simulink model "PubIfChassisAHBC_MDL"  (R2020b)
settings: Solver=FixedStepDiscrete  StartTime=0.0  StopTime=10.0  FixedStep=0.02  RelTol=1e-3
settings Model: DataDictionary=AHBC.sldd  Creator=mi  LastModifiedBy=GW00204750
settings OptimizationCC: DefaultParameterBehavior=Inlined  EnhancedBackFolding=on  PassReuseOutputArgsAs=Individual arguments  ZeroExternalMemoryAtStartup=off  ZeroInternalMemoryAtStartup=off  OptimizeBlockOrder=speed  DifferentSizesBufferReuse=on  OptimizationCustomize=off  EfficientTunableParamExpr=on
settings DebuggingCC: ParameterPrecisionLossMsg=none  ParameterTunabilityLossMsg=error  SFExecutionAtInitializationDiag=none  UnderSpecifiedDimensionMsg=warning  ArithmeticOperatorsInVariantConditions=warning
settings SFSimCC: MATLABDynamicMemAlloc=off  CustomCodeUndefinedFunction=UseInterfaceOnly
settings RTWCC: Description=Embedded Coder  SystemTargetFile=ert.tlc  TemplateMakefile=ert_default_tmf  GenerateReport=on  Toolchain=Microsoft Visual C++ 2019 v16.0 | nmake (64-bit Windows)  IncludeHyperlinkInReport=on  LaunchReport=on  GenerateTraceInfo=on  GenerateTraceReport=on  GenerateTraceReportSl=on  GenerateTraceReportSf=on  GenerateTraceReportEml=on
settings CodeAppCC: ForceParamTrailComments=on  IgnoreCustomStorageClasses=off  OperatorAnnotations=on  SimulinkDataObjDesc=on  SFDataObjDesc=on  InsertBlockDesc=on
settings ERTTargetCC: TargetLangStandard=C99 (ISO)  GenerateSampleERTMain=on  SupportNonFinite=off  SupportComplex=off  InlinedParameterPlacement=NonHierarchical  ERTCustomFileTemplate=example_file_process.tlc

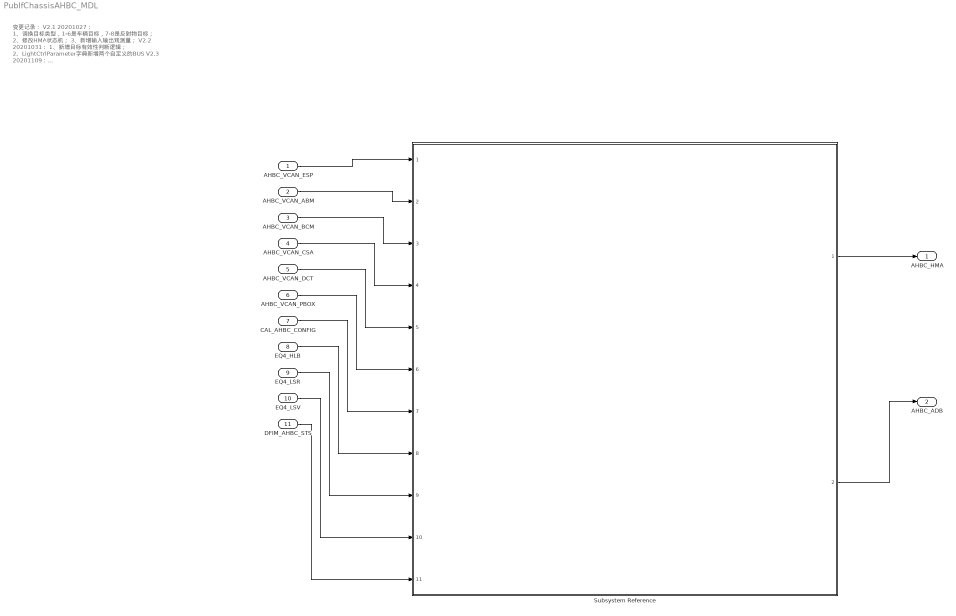
== system PubIfChassisAHBC_MDL ==
  note: 变更记录：
      | V2.1
      | 20201027：
      | 1、调换目标类型，1-6是车辆目标，7-8是反射物目标；
      | 2、修改HMA状态机；
      | 3、新增输入输出观测量；
      | V2.2
      | 20201031：
      | 1、新增目标有效性判断逻辑；
      | 2、LightCtrlParameter字典新增两个自定义的BUS
      | V2.3
      | 20201109：
      | 1、新增后雾灯RFogLmpSts__Pbox信号作为抑制条件；
      | 2、修复行驶方向抑制条件BUG；
      | V2.4
      | 20210104
      | 1、修复行驶方向抑制条件BUG；
      | 2、更改Trafficstyle命名为TrafficStyle
      |
      | 20210201
      | 1、匹配4.11DBC接口
      | 210217
      | 新增标定量P_AHBC_TrafficStyle，默认值为1；
      | 210218
      | 修复上电开始CamerSts报fault问题；
      | 210220
      | 优化AmBlight、RoadIllumDetd信号判断逻辑；
      | 210228
      | 增加目标跳变优化策略
      | 210301
      | 优化bug
      | 210302
      | 1、优化跳变bug
      | 2、修改有效性判断
      | 2010304
      | 优化AmBlight逻辑
      | 20210305
      | 优化BUG
      | 20210312
      | 屏蔽多余的目标有效性判断条件
  AHBC_VCAN_ESP : Inport  OutDataTypeStr=Bus: VCAN_ESP_MSG_BUS  PortDimensions=1  BusOutputAsStruct=on
  AHBC_VCAN_ABM : Inport  Port=2  OutDataTypeStr=Bus: VCAN_ABM_MSG_BUS  PortDimensions=1  BusOutputAsStruct=on
  AHBC_VCAN_BCM : Inport  Port=3  OutDataTypeStr=Bus: VCAN_BCM_MSG_BUS  PortDimensions=1  BusOutputAsStruct=on
  AHBC_VCAN_CSA : Inport  Port=4  OutDataTypeStr=Bus: VCAN_CSA_MSG_BUS  PortDimensions=1  BusOutputAsStruct=on
  AHBC_VCAN_DCT : Inport  Port=5  OutDataTypeStr=Bus: VCAN_DCT_MSG_BUS  PortDimensions=1  BusOutputAsStruct=on
  AHBC_VCAN_PBOX : Inport  Port=6  OutDataTypeStr=Bus: VCAN_PBOX_MSG_BUS  PortDimensions=1  BusOutputAsStruct=on
  CAL_AHBC_CONFIG : Inport  Port=7  OutDataTypeStr=Bus: CAL_AHBC_CONFIG_BUS  PortDimensions=1  BusOutputAsStruct=on
  EQ4_HLB : Inport  Port=8  OutDataTypeStr=Bus: EQ4_HLB_BUS  PortDimensions=1  BusOutputAsStruct=on
  EQ4_LSR : Inport  Port=9  OutDataTypeStr=Bus: EQ4_LSR_BUS  PortDimensions=1  BusOutputAsStruct=on
  EQ4_LSV : Inport  Port=10  OutDataTypeStr=Bus: EQ4_LSV_BUS  PortDimensions=1  BusOutputAsStruct=on
  DFIM_AHBC_STS : Inport  Port=11  OutDataTypeStr=Bus: DFIM_AHBC_STS_BUS  PortDimensions=1  BusOutputAsStruct=on
  Subsystem Reference : Subsystem  ReferencedSubsystem=PvtSubSys_AHBC
  AHBC_HMA : Outport  OutDataTypeStr=Bus: AHBC_HMA_BUS  PortDimensions=1  BusOutputAsStruct=on
  AHBC_ADB : Outport  Port=2  OutDataTypeStr=Bus: AHBC_ADB_BUS  PortDimensions=1  BusOutputAsStruct=on
  wires:
  AHBC_VCAN_ESP/1 -> Subsystem Reference/1
  AHBC_VCAN_ABM/1 -> Subsystem Reference/2
  AHBC_VCAN_BCM/1 -> Subsystem Reference/3
  AHBC_VCAN_CSA/1 -> Subsystem Reference/4
  AHBC_VCAN_DCT/1 -> Subsystem Reference/5
  AHBC_VCAN_PBOX/1 -> Subsystem Reference/6
  CAL_AHBC_CONFIG/1 -> Subsystem Reference/7
  EQ4_HLB/1 -> Subsystem Reference/8
  EQ4_LSR/1 -> Subsystem Reference/9
  EQ4_LSV/1 -> Subsystem Reference/10
  DFIM_AHBC_STS/1 -> Subsystem Reference/11
  Subsystem Reference/1 -> AHBC_HMA/1
  Subsystem Reference/2 -> AHBC_ADB/1
